simulink model "Deel2_volledig_oud"  (R2020b)
settings: Solver=FixedStepAuto  StartTime=0.0  StopTime=10.0  FixedStep=0.001  RelTol=1e-3  EnableMultiTasking=on
libraries: fl_lib x10, nesl_utility x4
settings Model: Creator=vande  LastModifiedBy=vande
settings SolverCC: PositivePriorityOrder=on
settings DataIOCC: ReturnWorkspaceOutputs=off
settings DebuggingCC: UnconnectedInputMsg=none  UnconnectedOutputMsg=none  UnconnectedLineMsg=none  SFMachineParentedDataDiag=error
settings ModelReferenceCC: EnableRefExpFcnMdlSchedulingChecks=off

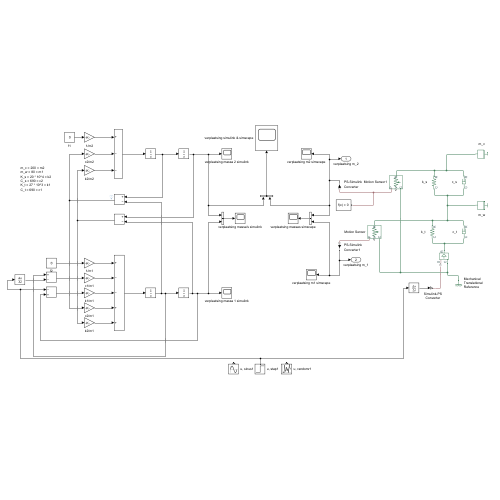
[thumbnail: Simulink's stored preview of the top-level diagram]
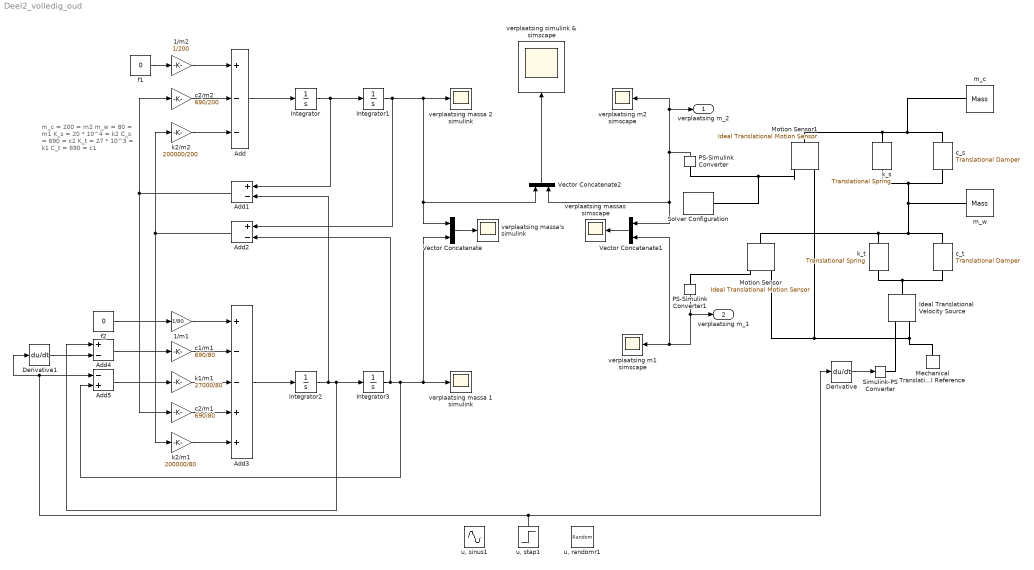
== system Deel2_volledig_oud ==
  note: m_c = 200 = m2
      | m_w = 80 = m1
      | K_s = 20 * 10^4 = k2
      | C_s = 690 = c2
      | K_t = 27 * 10^3 = k1
      | C_t = 690 = c1
  1/m1 : Gain  Gain=1/80
  1/m2 : Gain  Gain=1/200
  Add : Sum  Inputs=+--
  Add1 : Sum  Inputs=+-
  Add2 : Sum  Inputs=+-
  Add3 : Sum  Inputs=+--++
  Add4 : Sum  Inputs=+-
  Add5 : Sum  Inputs=-+
  Derivative : Derivative
  Derivative1 : Derivative
  Ideal Translational Velocity Source : fl_lib/Mechanical/Mechanical Sources/Ideal Translational Velocity Source
  Integrator{,1..3} (4 alike) : Integrator
  Mechanical Translational Reference : fl_lib/Mechanical/Translational Elements/Mechanical Translational Reference
  Motion Sensor : fl_lib/Mechanical/Mechanical Sensors/Ideal Translational Motion Sensor  reference=foundation.enum.MeasurementReference.difference  acceleration_port=false  velocity_port=true  position_port=true  offset=0 m
  Motion Sensor1 : fl_lib/Mechanical/Mechanical Sensors/Ideal Translational Motion Sensor  reference=foundation.enum.MeasurementReference.difference  acceleration_port=false  velocity_port=true  position_port=true  offset=0 m
  PS-Simulink Converter : nesl_utility/PS-Simulink Converter  PhysicalDomain=network_engine_domain  SubClassName=ps_output  LeftPortType=input  RightPortType=output  PseudoPeriodic=off  Frequencies=[]  VectorFormat=inherit  Unit=inherit  AffineConversion=off
  PS-Simulink Converter1 : nesl_utility/PS-Simulink Converter  PhysicalDomain=network_engine_domain  SubClassName=ps_output  LeftPortType=input  RightPortType=output  PseudoPeriodic=off  Frequencies=[]  VectorFormat=inherit  Unit=inherit  AffineConversion=off
  Simulink-PS Converter : nesl_utility/Simulink-PS Converter  PhysicalDomain=network_engine_domain  SubClassName=ps_input  LeftPortType=input  RightPortType=output  PseudoPeriodic=off  Frequencies=[]  NoiseDistribution=none  NoiseParameters=[]  Unit=1  AffineConversion=off  FilteringAndDerivatives=provide  SimscapeFilterOrder=1  InputFilterTimeConstant=0.001  UdotUserProvided=0
  Solver Configuration : nesl_utility/Solver Configuration  PhysicalDomain=network_engine_domain  SubClassName=solver  LeftPortType=input  RightPortType=generic  Tones=[]  Harmonics=[]  SimulateNoise=off  Profile=off  UseLocalSampling=off  EnableSwitchedLinearOptims=on  FrequencyDomain=off  UseCCode=off  RelTol=0.001  AbsTol=0.001  MinStep=1e-09  ToWorkspace=off  RevertToSquareIcSolve=off  NumHomotopyIterations=100  PhasorMode=off  PhasorModeNumHarmonics=1  ConsistencySolver=NEWTON_FTOL  IndexReductionMethod=DerivativeReplacement  DoDC=off  ResidualTolerance=1e-09  ConsistencyTolSource=GLOBAL  ConsistencyAbsTol=0.001  ConsistencyRelTol=0.001  ConsistencyTolFactor=0.001  UseLocalSolver=off  LocalSolverChoice=NE_BACKWARD_EULER_ADVANCER  ResolveIndetEquations=on  FunctionEvalNumThread=1  LocalSolverSampleTime=0.001  DoFixedCost=off  MaxNonlinIter=3  MaxModeIter=2  ComputeImpulses=off  ImpulseIterations=2  LinearAlgebra=auto  LinearAlgebraNumThread=0  EquationFormulation=NE_TIME_EF  DelaysMemoryBudget=1024  AutomaticFiltering=on  FilteringTimeConstant=0.001  PartitionStorageMethod=AS_NEEDED  PartitionMemoryBudget=1024  PartitionMethod=ROBUST
  Vector Concatenate : Concatenate
  Vector Concatenate1 : Concatenate
  Vector Concatenate2 : Concatenate
  c1/m1 : Gain  Gain=690/80
  c2/m1 : Gain  Gain=690/80
  c2/m2 : Gain  Gain=690/200
  c_s : fl_lib/Mechanical/Translational Elements/Translational Damper  D=690 N*s/m  v_specify=off  v_priority=None  v=0 m/s  v_nominal_specify=off  v_nominal_unit=m/s  v_nominal_value=1  f_specify=off  f_priority=None  f=0 N  f_nominal_specify=off  f_nominal_unit=N  f_nominal_value=1
  c_t : fl_lib/Mechanical/Translational Elements/Translational Damper  D=690 N*s/m  v_specify=off  v_priority=None  v=0 m/s  v_nominal_specify=off  v_nominal_unit=m/s  v_nominal_value=1  f_specify=off  f_priority=None  f=0 N  f_nominal_specify=off  f_nominal_unit=N  f_nominal_value=1
  f1 : Constant  Value=0
  f2 : Constant  Value=0
  k1/m1 : Gain  Gain=27000/80
  k2/m1 : Gain  Gain=200000/80
  k2/m2 : Gain  Gain=200000/200
  k_s : fl_lib/Mechanical/Translational Elements/Translational Spring  spr_rate=200000 N/m  v_specify=off  v_priority=None  v=0 m/s  v_nominal_specify=off  v_nominal_unit=m/s  v_nominal_value=1  f_specify=off  f_priority=None  f=0 N  f_nominal_specify=off  f_nominal_unit=N  f_nominal_value=1  x_specify=off  x_priority=High  x=0.1 m  x_nominal_specify=off  x_nominal_unit=m  x_nominal_value=1
  k_t : fl_lib/Mechanical/Translational Elements/Translational Spring  spr_rate=27000 N/m  v_specify=off  v_priority=None  v=0 m/s  v_nominal_specify=off  v_nominal_unit=m/s  v_nominal_value=1  f_specify=off  f_priority=None  f=0 N  f_nominal_specify=off  f_nominal_unit=N  f_nominal_value=1  x_specify=off  x_priority=High  x=0 m  x_nominal_specify=off  x_nominal_unit=m  x_nominal_value=1
  m_c : fl_lib/Mechanical/Translational Elements/Mass  mass=200 kg  num_ports=foundation.enum.numPorts2.one  v_specify=off  v_priority=High  v=0 m/s  v_nominal_specify=off  v_nominal_unit=m/s  v_nominal_value=1  f_specify=off  f_priority=None  f=0 N  f_nominal_specify=off  f_nominal_unit=N  f_nominal_value=1
  m_w : fl_lib/Mechanical/Translational Elements/Mass  mass=80 kg  num_ports=foundation.enum.numPorts2.one  v_specify=off  v_priority=High  v=0 m/s  v_nominal_specify=off  v_nominal_unit=m/s  v_nominal_value=1  f_specify=off  f_priority=None  f=0 N  f_nominal_specify=off  f_nominal_unit=N  f_nominal_value=1
  "u, randomr1" : UniformRandomNumber  Minimum=0  Maximum=0.02  SampleTime=0.01
  "u, sinus1" : Sin  Amplitude=0.02  Frequency=31.416  SampleTime=0
  "u, stap1" : Step  Time=5  After=0.05  SampleTime=0
  verplaatsing m1 simscape : Scope
  verplaatsing m2 simscape : Scope
  verplaatsing massa 1 simulink : Scope
  verplaatsing massa 2 simulink : Scope
  verplaatsing massa's simulink : Scope
  verplaatsing massas simscape : Scope
  verplaatsing simulink & simscape : Scope
  verplaatsing m_2 : Outport
  verplaatsing m_1 : Outport  Port=2
  wires:
  PS-Simulink Converter/1 -> Vector Concatenate1/1, Vector Concatenate2/2, verplaatsing m_2/1, verplaatsing m2 simscape/1
  PS-Simulink Converter1/1 -> verplaatsing m_1/1, verplaatsing m1 simscape/1, Vector Concatenate1/2
  Derivative/1 -> Simulink-PS Converter/1
  Integrator/1 -> Add1/1, Integrator1/1
  c2/m2/1 -> Add/2
  k2/m1/1 -> Add3/5
  k1/m1/1 -> Add3/3
  Add2/1 -> k2/m2/1, k2/m1/1
  1/m2/1 -> Add/1
  k2/m2/1 -> Add/3
  Integrator1/1 -> verplaatsing massa 2 simulink/1, Vector Concatenate2/1, Vector Concatenate/1, Add2/1
  Add5/1 -> k1/m1/1
  Integrator2/1 -> Add4/1, Integrator3/1, Add1/2
  Add/1 -> Integrator/1
  Add1/1 -> c2/m2/1, c2/m1/1
  1/m1/1 -> Add3/1
  f1/1 -> 1/m2/1
  c1/m1/1 -> Add3/2
  Add3/1 -> Integrator2/1
  c2/m1/1 -> Add3/4
  Derivative1/1 -> Add4/2
  Add4/1 -> c1/m1/1
  Integrator3/1 -> Add2/2, Add5/2, Vector Concatenate/2, verplaatsing massa 1 simulink/1
  f2/1 -> 1/m1/1
  Vector Concatenate/1 -> verplaatsing massa's simulink/1
  "u, stap1"/1 -> Derivative1/1, Add5/1, Derivative/1
  Vector Concatenate1/1 -> verplaatsing massas simscape/1
  Vector Concatenate2/1 -> verplaatsing simulink & simscape/1
  connections:
  k_s/LConn1 -- Motion Sensor1/LConn1 -- m_c/LConn1 -- c_s/LConn1
  k_t/LConn1 -- Motion Sensor/LConn1 -- c_t/LConn1 -- m_w/LConn1 -- c_s/RConn1 -- k_s/RConn1
  Motion Sensor/RConn1 -- Mechanical Translational Reference/LConn1 -- Ideal Translational Velocity Source/RConn2 -- Motion Sensor1/RConn1
  PS-Simulink Converter/LConn1 -- Motion Sensor1/RConn3 -- Solver Configuration/RConn1
  PS-Simulink Converter1/LConn1 -- Motion Sensor/RConn3
  c_t/RConn1 -- Ideal Translational Velocity Source/LConn1 -- k_t/RConn1
  Simulink-PS Converter/RConn1 -- Ideal Translational Velocity Source/RConn1
